simulink model "custom_tank_disturbance"  (R2024b)
settings: Solver=VariableStepAuto  StartTime=0.0  StopTime=600  RelTol=1e-3
values from neighbouring files (symbols this model uses):
  a = 0.16    [Double_tank_parameters.m]    (also in Double_tank_parameters_non_disturbed.m)
  A = 33    [Double_tank_parameters.m]    (also in Double_tank_parameters_non_disturbed.m)
  Alin = [-alpha, 0; alpha, -alpha]    [Double_tank_parameters.m]    (also in Double_tank_parameters_non_disturbed.m)
  Blin = [beta; 0]    [Double_tank_parameters.m]    (also in Double_tank_parameters_non_disturbed.m)
  Clin = [0, 1]    [Double_tank_parameters.m]    (also in Double_tank_parameters_non_disturbed.m)
  Dlin = 0    [Double_tank_parameters.m]    (also in Double_tank_parameters_non_disturbed.m)
  fSamplingTime = 1/fSamplingFrequency    (= 0.0125)    [Double_tank_parameters.m]    (also in Double_tank_parameters_non_disturbed.m)
  g = 982    [Double_tank_parameters.m]    (also in Double_tank_parameters_non_disturbed.m)
  h = 15    [Double_tank_parameters.m]    (also in Double_tank_parameters_non_disturbed.m)
  h0 = 3.2    [Double_tank_parameters.m]    (also in Double_tank_parameters_non_disturbed.m)
  KgainC = Clin'*(Clin*PC*Clin' + R2)    [Double_tank_parameters_non_disturbed.m]
  Kkgain = Ccd'*(Ccd*Pp* Ccd' + R2)    [Double_tank_parameters.m]
  NN = eye(3,3)    [Double_tank_parameters.m]
  p1 = polyfit(u0, fu0, 3)    [Double_tank_parameters.m]    (also in Double_tank_parameters_non_disturbed.m)
  Qqd = eye(3,3)*0.01    [Double_tank_parameters.m]
  Rrd = R2    (= 0.01)    [Double_tank_parameters.m]
  u_h = r(n)    [Double_tank_parameters.m]    (also in Double_tank_parameters_non_disturbed.m)
undefined symbols (not defined in the file or in its folder): Aad, Bbd, Ccd, Pp
libraries: simulink x2, SignalEditorBlockLib x2
settings Model: Creator=beckl  LastModifiedBy=beckl

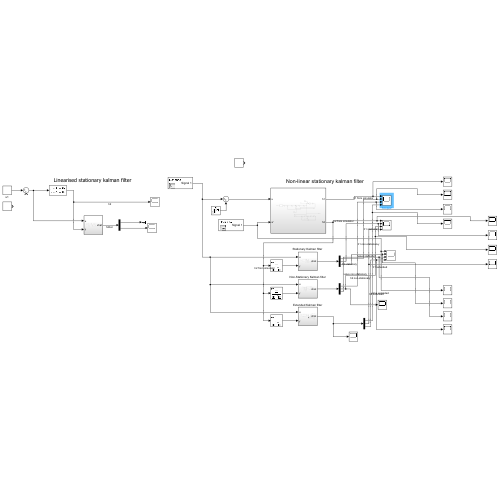
[thumbnail: Simulink's stored preview of the top-level diagram]
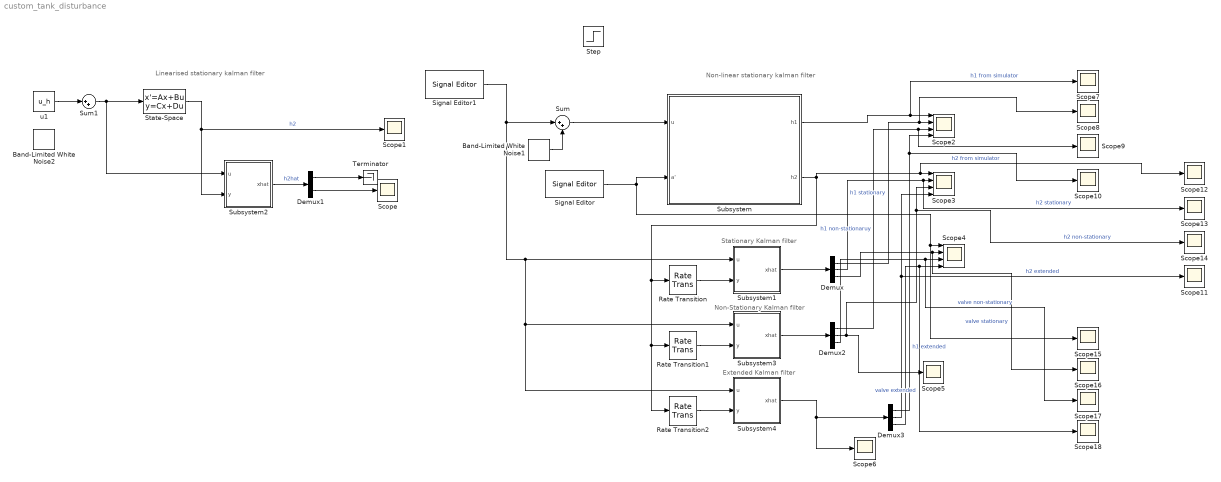
== system custom_tank_disturbance ==
  note: Non-Stationary Kalman filter
  note: Extended Kalman filter
  note: Stationary Kalman filter
  note: Linearised stationary kalman filter
  note: Non-linear stationary kalman filter
  Band-Limited White Noise1 : simulink/Sources/Band-Limited White Noise  Cov=[0.01]  Ts=fSamplingTime  seed=[23341]
  Band-Limited White Noise2 : simulink/Sources/Band-Limited White Noise  Cov=[0.1]  Ts=0.1  seed=[23341]
  Demux : Demux  Outputs=3
  Demux1 : Demux  Outputs=2
  Demux2 : Demux  Outputs=3
  Demux3 : Demux  Outputs=3
  Rate Transition : RateTransition  OutPortSampleTime=fSamplingTime
  Rate Transition1 : RateTransition  OutPortSampleTime=fSamplingTime
  Rate Transition2 : RateTransition  OutPortSampleTime=fSamplingTime
  Scope{,1,5..18} (16 alike) : Scope
  Scope2 : Scope  NumInputPorts=4
  Scope3 : Scope  NumInputPorts=4
  Scope4 : Scope  NumInputPorts=4
  Signal Editor : SignalEditorBlockLib/Signal Editor  FileName=C:\Users\beckl\OneDrive\Skrivbord\Kurser\R7014E Avancerade Reglersystem\Lab A\R7014E_lib_R003\R7014E_lib_R003\valve_opening.mat  ActiveScenario=Scenario  ActiveSignal=Signal 1  IsBus=off  OutputBusObjectStr=Bus: BusObject  SampleTime=0  Interpolate=off  ZeroCross=off  OutputAfterFinalValue=Setting to zero  Unit=inherit  PreserveSignalName=on  ApplySigPropsToAllScenarios=on  ApplySigPropsToAllSignals=off
  Signal Editor1 : SignalEditorBlockLib/Signal Editor  FileName=C:\Users\beckl\OneDrive\Skrivbord\Kurser\R7014E Avancerade Reglersystem\Lab A\R7014E_lib_R003\R7014E_lib_R003\voltage.mat  ActiveScenario=Scenario  ActiveSignal=Signal 1  IsBus=off  OutputBusObjectStr=Bus: BusObject  SampleTime=0  Interpolate=off  ZeroCross=off  OutputAfterFinalValue=Setting to zero  Unit=inherit  PreserveSignalName=on  ApplySigPropsToAllScenarios=on  ApplySigPropsToAllSignals=off
  State-Space : StateSpace  A=Alin  B=Blin  C=Clin  D=Dlin  InitialCondition=0
  Step : Step  Time=100  After=u_h  SampleTime=0
  Subsystem : Subsystem
  Subsystem1 : Subsystem
  Subsystem2 : Subsystem
  Subsystem3 : Subsystem
  Subsystem4 : Subsystem
  Sum : Sum  Inputs=|++
  Sum1 : Sum  Inputs=|++
  Terminator : Terminator
  u1 : Constant  Value=u_h
  wires:
  Sum/1 -> Subsystem/1(u)
  Subsystem/2(h2) -> Rate Transition2/1, Rate Transition1/1, Rate Transition/1, Scope12/1, Scope3/1  "h2 from simulator"
  Signal Editor1/1 -> Subsystem4/1(u), Subsystem3/1(u), Subsystem1/1(u), Sum/1
  u1/1 -> Sum1/1
  Sum1/1 -> Subsystem2/1(u), State-Space/1
  Rate Transition/1 -> Subsystem1/2(y)
  State-Space/1 -> Scope1/1, Subsystem2/2(y)  "h2"
  Subsystem2/1(xhat) -> Demux1/1  "h2hat"
  Demux1/1 -> Terminator/1
  Demux1/2 -> Scope/1
  Rate Transition1/1 -> Subsystem3/2(y)
  Band-Limited White Noise1/1 -> Sum/2
  Subsystem/1(h1) -> Scope7/1, Scope2/1  "h1 from simulator"
  Subsystem1/1(xhat) -> Demux/1
  Subsystem3/1(xhat) -> Demux2/1
  Demux/1 -> Scope8/1, Scope2/2  "h1 stationary"
  Demux/3 -> Scope16/1, Scope4/2  "valve stationary"
  Demux2/1 -> Scope9/1, Scope2/3  "h1 non-stationaruy"
  Demux2/2 -> Scope5/1, Scope3/3, Scope14/1  "h2 non-stationary"
  Demux2/3 -> Scope17/1, Scope4/3  "valve non-stationary"
  Demux/2 -> Scope13/1, Scope3/2  "h2 stationary"
  Signal Editor/1 -> Scope15/1, Scope4/1, Subsystem/2(a')
  Rate Transition2/1 -> Subsystem4/2(y)
  Subsystem4/1(xhat) -> Demux3/1, Scope6/1
  Demux3/1 -> Scope10/1, Scope2/4  "h1 extended"
  Demux3/2 -> Scope11/1, Scope3/4  "h2 extended"
  Demux3/3 -> Scope18/1, Scope4/4  "valve extended"

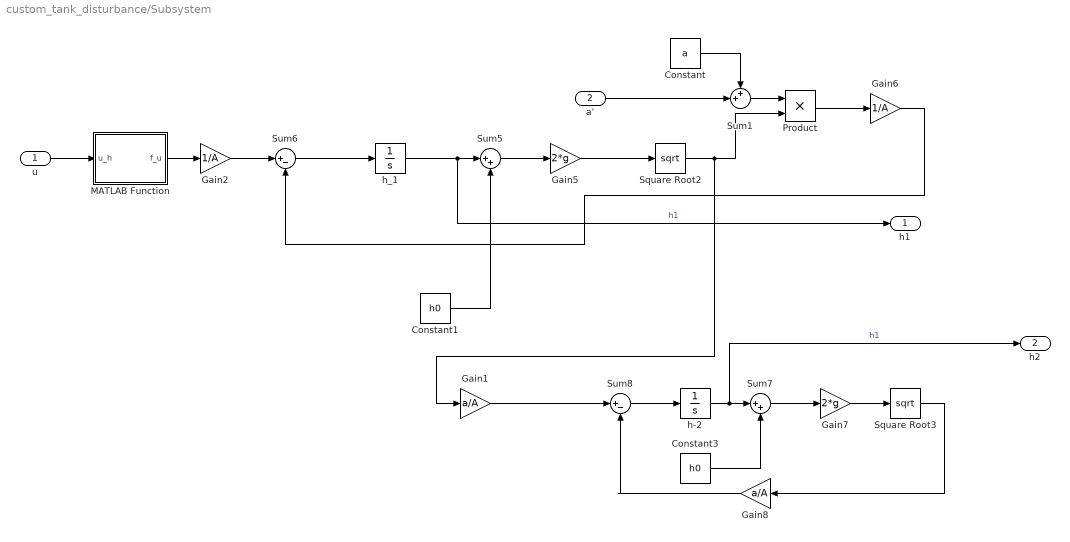
== system custom_tank_disturbance/Subsystem ==
  u : Inport
  a' : Inport  Port=2
  Constant : Constant  Value=a
  Constant1 : Constant  Value=h0
  Constant3 : Constant  Value=h0
  Gain1 : Gain  Gain=a/A
  Gain2 : Gain  Gain=1/A
  Gain5 : Gain  Gain=2*g
  Gain6 : Gain  Gain=1/A
  Gain7 : Gain  Gain=2*g
  Gain8 : Gain  Gain=a/A
  MATLAB Function : MATLAB Function  TreatAsAtomicUnit=on
  Product : Product
  Square Root2 : Sqrt
  Square Root3 : Sqrt
  Sum1 : Sum  Inputs=++|
  Sum5 : Sum  Inputs=|++
  Sum6 : Sum  Inputs=|+-
  Sum7 : Sum  Inputs=|++
  Sum8 : Sum  Inputs=|+-
  h-2 : Integrator
  h_1 : Integrator
  h1 : Outport
  h2 : Outport  Port=2
  wires:
  Square Root2/1 -> Gain1/1, Product/2
  Sum6/1 -> h_1/1
  Constant/1 -> Sum1/1
  Sum1/1 -> Product/1
  Square Root3/1 -> Gain8/1
  Gain6/1 -> Sum6/2
  Sum8/1 -> h-2/1
  h_1/1 -> h1/1, Sum5/1  "h1"
  Gain2/1 -> Sum6/1
  Product/1 -> Gain6/1
  Gain5/1 -> Square Root2/1
  MATLAB Function/1(f_u) -> Gain2/1
  Sum5/1 -> Gain5/1
  u/1 -> MATLAB Function/1(u_h)
  Constant1/1 -> Sum5/2
  Sum7/1 -> Gain7/1
  Gain7/1 -> Square Root3/1
  a'/1 -> Sum1/2
  h-2/1 -> h2/1, Sum7/1  "h1"
  Constant3/1 -> Sum7/2
  Gain8/1 -> Sum8/2
  Gain1/1 -> Sum8/1

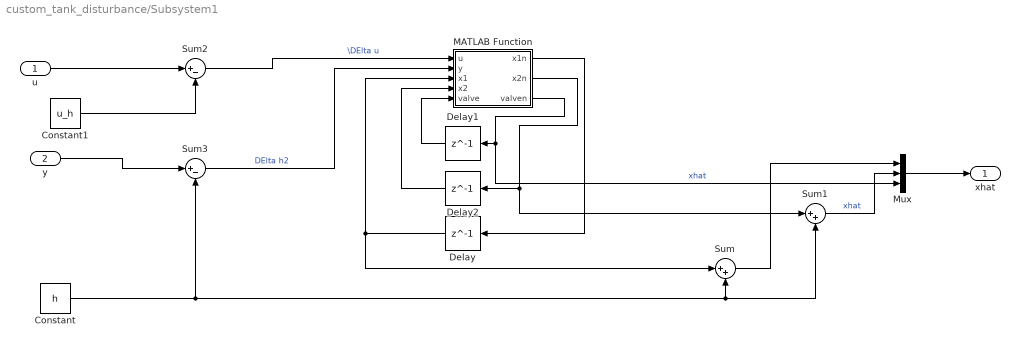
== system custom_tank_disturbance/Subsystem1 ==
  u : Inport
  y : Inport  Port=2
  Constant : Constant  Value=h
  Constant1 : Constant  Value=u_h
  Delay : Delay  DelayLength=1  InitialCondition=0  SampleTime=fSamplingTime
  Delay1 : Delay  DelayLength=1  InitialCondition=0  SampleTime=fSamplingTime
  Delay2 : Delay  DelayLength=1  InitialCondition=0  SampleTime=fSamplingTime
  MATLAB Function : MATLAB Function  TreatAsAtomicUnit=on
  Mux : Mux  Inputs=3
  Sum : Sum  Inputs=|++
  Sum1 : Sum  Inputs=|++
  Sum2 : Sum  Inputs=|+-
  Sum3 : Sum  Inputs=|+-
  xhat : Outport
  wires:
  Constant1/1 -> Sum2/2
  u/1 -> Sum2/1
  y/1 -> Sum3/1
  Sum3/1 -> MATLAB Function/2(y)  "DElta h2"
  Sum2/1 -> MATLAB Function/1(u)  "\\DElta u"
  Delay/1 -> Sum/1, MATLAB Function/3(x1)
  MATLAB Function/1(x1n) -> Delay/1
  MATLAB Function/2(x2n) -> Sum1/1, Delay2/1
  Delay2/1 -> MATLAB Function/4(x2)
  Delay1/1 -> MATLAB Function/5(valve)
  Mux/1 -> xhat/1
  MATLAB Function/3(valven) -> Mux/3, Delay1/1  "xhat"
  Sum1/1 -> Mux/2  "xhat"
  Sum/1 -> Mux/1
  Constant/1 -> Sum1/2, Sum/2, Sum3/2

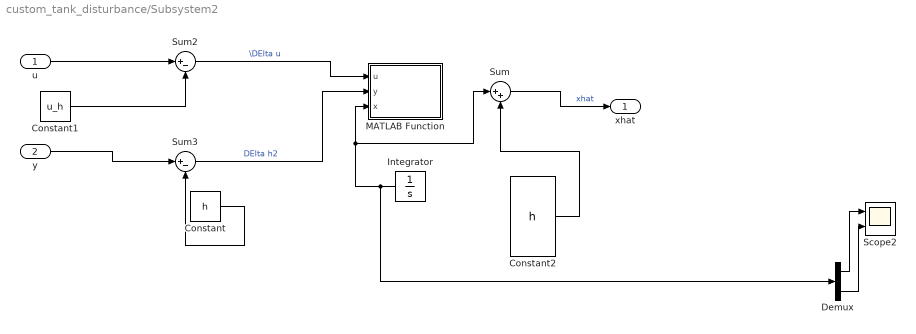
== system custom_tank_disturbance/Subsystem2 ==
  u : Inport
  y : Inport  Port=2
  Constant : Constant  Value=h
  Constant1 : Constant  Value=u_h
  Constant2 : Constant  Value=h
  Demux : Demux  Outputs=2
  Integrator : Integrator
  MATLAB Function : MATLAB Function  TreatAsAtomicUnit=on
  Scope2 : Scope  NumInputPorts=2
  Sum : Sum  Inputs=|++
  Sum2 : Sum  Inputs=|+-
  Sum3 : Sum  Inputs=|+-
  xhat : Outport
  wires:
  Constant/1 -> Sum3/2
  u/1 -> Sum2/1
  y/1 -> Sum3/1
  Sum/1 -> xhat/1  "xhat"
  Sum3/1 -> MATLAB Function/2(y)  "DElta h2"
  Sum2/1 -> MATLAB Function/1(u)  "\\DElta u"
  Integrator/1 -> Demux/1, Sum/1, MATLAB Function/3(x)
  Constant2/1 -> Sum/2
  ? -> Integrator/1
  Demux/2 -> Scope2/2
  Demux/1 -> Scope2/1
  Constant1/1 -> Sum2/2

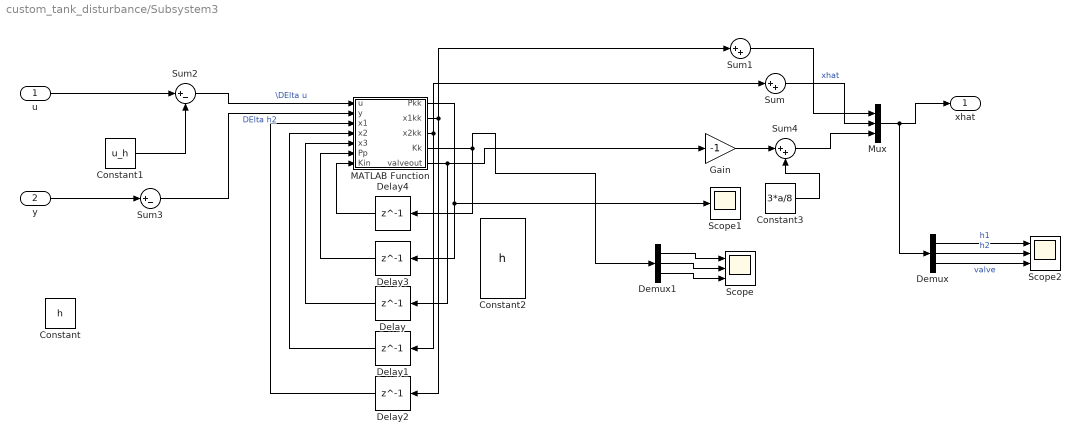
== system custom_tank_disturbance/Subsystem3 ==
  u : Inport
  y : Inport  Port=2
  Constant : Constant  Value=h
  Constant1 : Constant  Value=u_h
  Constant2 : Constant  Value=h
  Constant3 : Constant  Value=3*a/8
  Delay : Delay  DelayLength=1
  Delay1 : Delay  DelayLength=1
  Delay2 : Delay  DelayLength=1
  Delay3 : Delay  DelayLength=1  InitialCondition=Pp
  Delay4 : Delay  DelayLength=1  InitialCondition=[0;0;0]
  Demux : Demux  Outputs=3
  Demux1 : Demux  Outputs=3
  Gain : Gain  Gain=-1
  MATLAB Function : MATLAB Function  TreatAsAtomicUnit=on
  Mux : Mux  Inputs=3
  Scope : Scope  NumInputPorts=3
  Scope1 : Scope
  Scope2 : Scope  NumInputPorts=3
  Sum : Sum  Inputs=|++
  Sum1 : Sum  Inputs=|++
  Sum2 : Sum  Inputs=|+-
  Sum3 : Sum  Inputs=|+-
  Sum4 : Sum  Inputs=|++
  xhat : Outport
  wires:
  Constant1/1 -> Sum2/2
  u/1 -> Sum2/1
  Sum3/1 -> MATLAB Function/2(y)  "DElta h2"
  Sum2/1 -> MATLAB Function/1(u)  "\\DElta u"
  MATLAB Function/1(Pkk) -> Scope1/1, Delay3/1
  MATLAB Function/2(x1kk) -> Sum1/1, Delay2/1
  MATLAB Function/3(x2kk) -> Sum/1, Delay1/1
  MATLAB Function/5(valveout) -> Gain/1, Delay/1
  Sum1/1 -> Mux/1
  Sum/1 -> Mux/2  "xhat"
  Mux/1 -> Demux/1, xhat/1
  Delay2/1 -> MATLAB Function/3(x1)
  Delay1/1 -> MATLAB Function/4(x2)
  Delay/1 -> MATLAB Function/5(x3)
  Delay3/1 -> MATLAB Function/6(Pp)
  y/1 -> Sum3/1
  Demux/3 -> Scope2/3  "valve"
  Demux/1 -> Scope2/1  "h1"
  Demux/2 -> Scope2/2  "h2"
  Demux1/1 -> Scope/1
  Demux1/2 -> Scope/2
  Demux1/3 -> Scope/3
  MATLAB Function/4(Kk) -> Demux1/1, Delay4/1
  Delay4/1 -> MATLAB Function/7(Kin)
  Gain/1 -> Sum4/1
  Sum4/1 -> Mux/3
  Constant3/1 -> Sum4/2

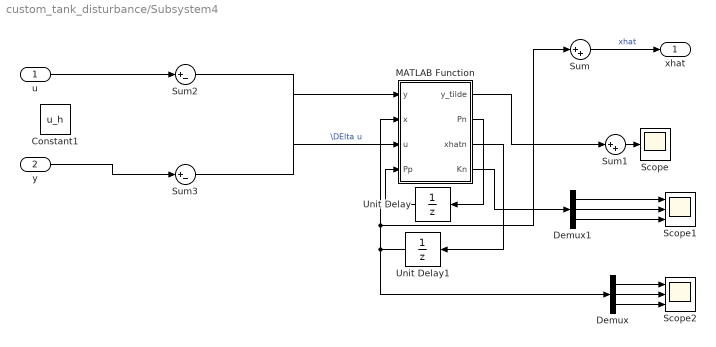
== system custom_tank_disturbance/Subsystem4 ==
  u : Inport
  y : Inport  Port=2
  Constant1 : Constant  Value=u_h
  Demux : Demux  Outputs=3
  Demux1 : Demux  Outputs=3
  MATLAB Function : MATLAB Function  TreatAsAtomicUnit=on
  Scope : Scope
  Scope1 : Scope  NumInputPorts=3
  Scope2 : Scope  NumInputPorts=3
  Sum : Sum  Inputs=|++
  Sum1 : Sum  Inputs=|++
  Sum2 : Sum  Inputs=|+-
  Sum3 : Sum  Inputs=|+-
  Unit Delay : UnitDelay  InitialCondition=Pp  SampleTime=-1  HasFrameUpgradeWarning=on
  Unit Delay1 : UnitDelay  InitialCondition=[0;0;0]  SampleTime=-1  HasFrameUpgradeWarning=on
  xhat : Outport
  wires:
  Demux1/1 -> Scope1/1
  Demux1/2 -> Scope1/2
  MATLAB Function/4(Kn) -> Demux1/1
  MATLAB Function/1(y_tilde) -> Sum1/1
  MATLAB Function/3(xhatn) -> Unit Delay1/1
  Sum1/1 -> Scope/1
  Sum/1 -> xhat/1  "xhat"
  Demux/1 -> Scope2/1
  Sum3/1 -> MATLAB Function/1(y)
  Sum2/1 -> MATLAB Function/3(u)  "\\DElta u"
  y/1 -> Sum3/1
  Unit Delay1/1 -> MATLAB Function/2(x), Sum/1, Demux/1
  u/1 -> Sum2/1
  Unit Delay/1 -> MATLAB Function/4(Pp)
  MATLAB Function/2(Pn) -> Unit Delay/1
  Demux/2 -> Scope2/2
  Demux1/3 -> Scope1/3
  Demux/3 -> Scope2/3

== matlab function custom_tank_disturbance/Subsystem4/MATLAB Function ==
  data: y input; x input; y_tilde output; Pn output; u input; Pp input; p1 parameter; xhatn output; Qqd parameter; Rrd parameter; Kn output; h parameter
function [y_tilde, Pn, xhatn, Kn] = fcn(y, x, u, Pp, p1, Qqd, Rrd, h)

fSamplingFrequency = 80;
fSamplingTime = 1/fSamplingFrequency;
A = 33; % 33 square centimetres
a = 0.16; % 0.16 square centimetres
%T = 35; % 35 seconds time constant
%K = 5; % metres per volt, motor gain
h0 = 3.2;
g = 982;


% Linearise around current point
% if x(1) + h0 < 0.01
%     x1 = 0.01;
% else
%     x1 = x(1) + h0;
% end
% 
% if x(2) + h0 < 0.01
%     x2 = 0.01;
% else
%     x2 = x(2) + h0;
% end

alpha1 = g*a/(A*sqrt(2*g*(x(1) + h0)));
alpha2 = g*a/(A*sqrt(2*g*(x(2) + h0)));
zeta = 1/A * sqrt(2*g*(x(1) + h0));

%error in linearisation
A1 = [-alpha1, 0, zeta; alpha1, alpha2, 0; 0, 0, 0];

%fixed linearisation
sqrt1 = sqrt(2*g*(x(1) + h0));
sqrt2 = sqrt(2*g*(x(1) + h0));

A1 = zeros(3, 3);
A1(1, 1) = -(a + x(3))/A * g/sqrt1;
A1(1, 3) = -1/A * sqrt1;
A1(2, 1) = a/A * g/sqrt1;
A1(2, 2) = -a/A * g/sqrt2;
An = eye(size(A1)) + fSamplingTime*A1;
Cn = [0, 1, 0];



% predict
q = p1(1)*u^3 + p1(2)*u^2 + p1(3)*u + p1(4);
xhatdot = [q/A-a/A*(sqrt(2*g*(x(1) + h0)))-x(3)/A*sqrt(2*g*(x(1) + h0));
    a/A*(sqrt(2*g*(x(1) + h0)))-a/A*(sqrt(2*g*(x(2) + h0)));
    0];
xhatn = x + xhatdot.*fSamplingTime;
Pn = An * Pp * An' + Qqd;

% update
y_tilde = y - Cn * xhatn;
S = Cn * Pn * Cn'+ Rrd;
Kn = S\(Pn * Cn');
xhatn = xhatn + Kn*y_tilde;
Pn = (eye(size(An)) - Kn*Cn)*Pn;
y_tilde = y - Cn*xhatn;

== matlab function custom_tank_disturbance/Subsystem1/MATLAB Function ==
  data: u input; x1n output; y input; x1 input; x2 input; valve input; Aad parameter; Bbd parameter; Ccd parameter; Kkgain parameter; x2n output; valven output
function [x1n, x2n, valven] = fcn(u,y,x1, x2, valve,Aad, Bbd, Ccd, Kkgain)
x=[x1;x2;valve];
% xn = [0;0;0];
xn =Aad*x+Bbd*u+Kkgain*(y-Ccd*x);
x1n = xn(1);
x2n = xn(2);
valven = xn(3);

== matlab function custom_tank_disturbance/Subsystem/MATLAB Function ==
  data: u_h input; f_u output; p1 parameter
function f_u = fcn(u_h,p1)
f_u  = polyval(p1, u_h);;

== matlab function custom_tank_disturbance/Subsystem2/MATLAB Function ==
  data: u input; y input; x input; Alin parameter; Blin parameter; Clin parameter; KgainC parameter
function fcn(u,y,x,Alin, Blin, Clin, KgainC)
xn=[0;0];
xn =Alin*x+Blin*u+KgainC*(y-Clin*x);

== matlab function custom_tank_disturbance/Subsystem3/MATLAB Function ==
  data: Pkk output; u input; x1kk output; y input; x1 input; x2 input; x3 input; Aad parameter; Bbd parameter; Ccd parameter; Qqd parameter; Rrd parameter; Pp input; NN parameter; x2kk output; Kk output; valveout output; Kin input
% function [Pkk, x1kk, x2kk, Kk, valveout] = fcn(u,y,x1, x2, x3, Aad, Bbd, Ccd, Qqd, Rrd, Pp, NN, Kin)
% %xn =Ad*x+Bd*u+Kgain*(y-Cd*x); %stationary
% %xn = Ad*x + Bd*u + N*v;
% % Sk = 0
% 
%     x = [x1;x2;x3];
%     xk = Aad*x + Bbd*u;
%     Pk = Aad*Pp*Aad' + NN*Qqd*NN';
%     %Pk = cov(x, xk);
% 
%     % determine current kalman gain
% 
%     y_tilde = y-Ccd*xk;
% 
%     xkk = xk + Kin*y_tilde;
%     Pkk = Pk - Kin*Ccd*Pk;
%     Kk = (Ccd*Pkk*Ccd'+Rrd)\(Pkk*Ccd');
%     x1kk = xkk(1);
%     x2kk = xkk(2);
%     valveout = xkk(3);

% function [Pkk, x1kk, x2kk, Kk, valveout] = fcn(u, y, x1, x2, x3, Aad, Bbd, Ccd, Qqd, Rrd, Pp, NN, Kin)
% % Non-stationary Kalman filter for leak estimation with smooth transitions
% % States: [water level; outflow; valve opening/leak]
% 
%     % Combine previous states
%     x = [x1; x2; x3];
% 
%     % --- Time update (prediction) ---
%     % A-priori state estimate
%     xk = Aad * x + Bbd * u;
% 
%     % A-priori error covariance
%     Pk = Aad * Pp * Aad' + NN * Qqd * NN';
% 
%     % --- Kalman gain calculation ---
%     % Innovation covariance
%     Sk = Ccd * Pk * Ccd' + Rrd;
% 
%     % Kalman gain
%     Kk = Sk \ Pk * Ccd';
% 
%     % --- Measurement update (correction) ---
%     % Innovation
%     y_tilde = y - Ccd * xk;
% 
%     % A-posteriori state estimate
%     xkk = xk + Kk * y_tilde;
% 
%     % A-posteriori error covariance
%     Pkk = (eye(size(Aad)) - Kk * Ccd) * Pk;
% 
%     % Extract states
%     x1kk = xkk(1);  % Water level
%     x2kk = xkk(2);  % Outflow
%     valveout = xkk(3);  % Leak opening (will track ramps naturally)
% 
% end

% trial 3
function [Pkk, x1kk, x2kk, Kk, valveout] = fcn(u,y,x1, x2, x3, Aad, Bbd, Ccd, Qqd, Rrd, Pp, NN, Kin)

xhat = [x1, x2, x3]';
% Sk = 0

xk1k = Aad*xhat + Bbd*u;
Pk1k = Aad*Pp*Aad' + NN*Qqd*NN';

Kk = (Ccd*Pk1k*Ccd' + Rrd)\Pk1k*Ccd';
y_tilde = y - Ccd*xk1k;
xk1k1 = xk1k + Kk*y_tilde;
Pk1k1 = Pk1k - Kk*Ccd*Pk1k;

Pkk = Pk1k1;
x1kk = xk1k1(1);
x2kk = xk1k1(2);
valveout = xk1k1(3);
